simulink library "hysteresis_curve"  (R2016b)
settings: Solver=VariableStepAuto  StartTime=0.0  StopTime=10.0  RelTol=1e-3
undefined symbols (not defined in the file or in its folder): sim_params
settings Model: Creator=bijan  LastModifiedBy=scrice

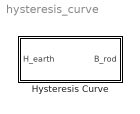
== system hysteresis_curve ==
  Hysteresis Curve : Subsystem

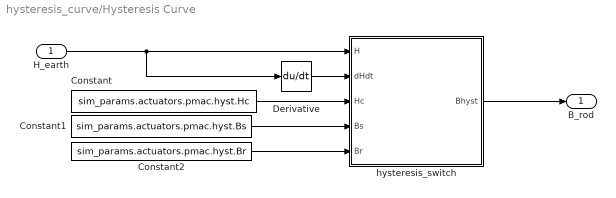
== system hysteresis_curve/Hysteresis Curve ==
  H_earth : Inport
  Constant : Constant  Value=sim_params.actuators.pmac.hyst.Hc
  Constant1 : Constant  Value=sim_params.actuators.pmac.hyst.Bs
  Constant2 : Constant  Value=sim_params.actuators.pmac.hyst.Br
  Derivative : Derivative
  hysteresis_switch : MATLAB Function  TreatAsAtomicUnit=on
  B_rod : Outport
  wires:
  Derivative/1 -> hysteresis_switch/2(dHdt)
  hysteresis_switch/1(Bhyst) -> B_rod/1
  Constant2/1 -> hysteresis_switch/5(Br)
  Constant1/1 -> hysteresis_switch/4(Bs)
  Constant/1 -> hysteresis_switch/3(Hc)
  H_earth/1 -> hysteresis_switch/1(H), Derivative/1

== matlab function hysteresis_curve/Hysteresis Curve/hysteresis_switch ==
  data: H input; Bhyst output; dHdt input; Hc input; Bs input; Br input
function Bhyst = fcn(H, dHdt, Hc, Bs, Br)
    if(dHdt >= 0)
        p = (1/Hc)*tan(pi*Br/(2*Bs));
        Bhyst = (2/pi)*Bs*atan(p*(H-Hc));
    else
        p = (1/Hc)*tan(pi*Br/(2*Bs));
        Bhyst = (2/pi)*Bs*atan(p*(H+Hc));
    end
end
